simulink model "ModeloControlador2"  (R2018a)
settings: Solver=VariableStepAuto  StartTime=0.0  StopTime=20  RelTol=1e-3
values from neighbouring files (symbols this model uses):
  grav = 9.81    [modelodrone.m]
  Jr = .00006    (= 6e-05)    [modelodrone.m]
  massa = 1.24706    [modelodrone.m]
undefined symbols (not defined in the file or in its folder): Drone
libraries: simulink x6
settings Model: Creator=lg07j  LastModifiedBy=lg07j

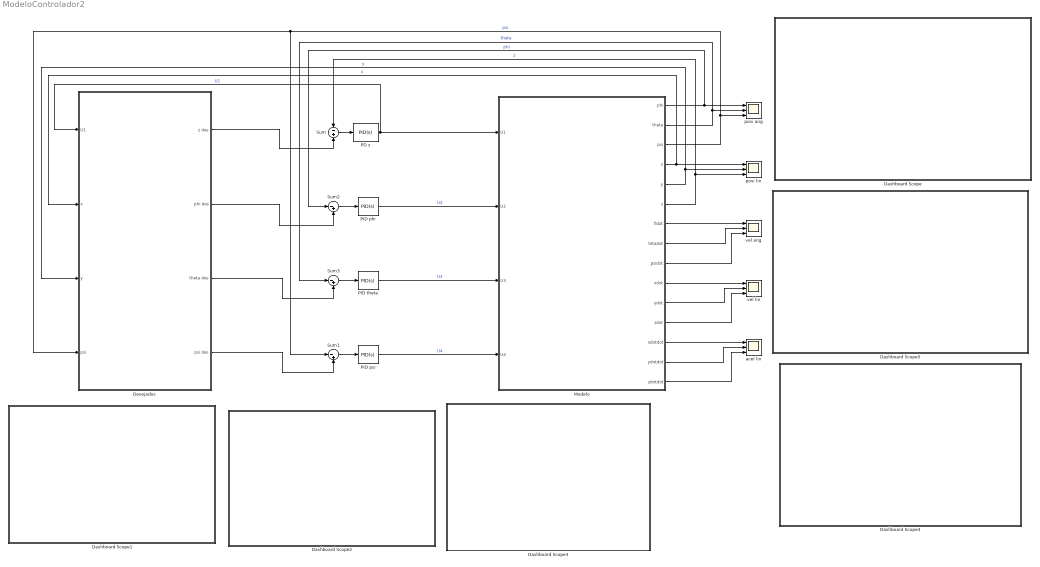
== system ModeloControlador2 ==
  Dashboard Scope : Subsystem  DialogController=hmiCreateDDGDialog  IsWebBlock=on  mask(MWDashboardBlock){webBlockId=ccebd60a-0072-45fe-991e-5f1cde7eeb39, webBlockType=sdiscope, ShowInitialText=on, HMISrcModelName=ModeloControlador2}
      mask prompts: webBlockId "WebBlock Id"; webBlockType "WebBlock Type"; HMISrcModelName "Source Model"
      mask help: SimulinkHMI:dialogs:HMIScopeDialogDesc
      mask Help: helpview([docroot '/mapfiles/simulink.map'], 'hmi_scope')
      mask Display:
      | if strcmp(get_param(bdroot(gcb),'BlockDiagramType'), 'library')
      |     image([(matlabroot) '/toolbox/simulink/hmi/icons/DashboardScope.png']);
      | end
  Dashboard Scope1 : Subsystem  DialogController=hmiCreateDDGDialog  IsWebBlock=on  mask(MWDashboardBlock){webBlockId=5c128209-e94a-417c-b40b-eaa209d18782, webBlockType=sdiscope, ShowInitialText=on, HMISrcModelName=ModeloControlador2}
      mask prompts: webBlockId "WebBlock Id"; webBlockType "WebBlock Type"; HMISrcModelName "Source Model"
      mask help: SimulinkHMI:dialogs:HMIScopeDialogDesc
      mask Help: helpview([docroot '/mapfiles/simulink.map'], 'hmi_scope')
      mask Display:
      | if strcmp(get_param(bdroot(gcb),'BlockDiagramType'), 'library')
      |     image([(matlabroot) '/toolbox/simulink/hmi/icons/DashboardScope.png']);
      | end
  Dashboard Scope2 : Subsystem  DialogController=hmiCreateDDGDialog  IsWebBlock=on  mask(MWDashboardBlock){webBlockId=3c2bd112-e6fb-4389-a652-d4a52c948602, webBlockType=sdiscope, ShowInitialText=on, HMISrcModelName=ModeloControlador2}
      mask prompts: webBlockId "WebBlock Id"; webBlockType "WebBlock Type"; HMISrcModelName "Source Model"
      mask help: SimulinkHMI:dialogs:HMIScopeDialogDesc
      mask Help: helpview([docroot '/mapfiles/simulink.map'], 'hmi_scope')
      mask Display:
      | if strcmp(get_param(bdroot(gcb),'BlockDiagramType'), 'library')
      |     image([(matlabroot) '/toolbox/simulink/hmi/icons/DashboardScope.png']);
      | end
  Dashboard Scope3 : Subsystem  DialogController=hmiCreateDDGDialog  IsWebBlock=on  mask(MWDashboardBlock){webBlockId=80d6d028-651e-447f-a397-777ee9cde126, webBlockType=sdiscope, ShowInitialText=on, HMISrcModelName=ModeloControlador2}
      mask prompts: webBlockId "WebBlock Id"; webBlockType "WebBlock Type"; HMISrcModelName "Source Model"
      mask help: SimulinkHMI:dialogs:HMIScopeDialogDesc
      mask Help: helpview([docroot '/mapfiles/simulink.map'], 'hmi_scope')
      mask Display:
      | if strcmp(get_param(bdroot(gcb),'BlockDiagramType'), 'library')
      |     image([(matlabroot) '/toolbox/simulink/hmi/icons/DashboardScope.png']);
      | end
  Dashboard Scope4 : Subsystem  DialogController=hmiCreateDDGDialog  IsWebBlock=on  mask(MWDashboardBlock){webBlockId=8646fb84-920d-4198-92bb-6f16b9d3f7b0, webBlockType=sdiscope, ShowInitialText=on, HMISrcModelName=ModeloControlador2}
      mask prompts: webBlockId "WebBlock Id"; webBlockType "WebBlock Type"; HMISrcModelName "Source Model"
      mask help: SimulinkHMI:dialogs:HMIScopeDialogDesc
      mask Help: helpview([docroot '/mapfiles/simulink.map'], 'hmi_scope')
      mask Display:
      | if strcmp(get_param(bdroot(gcb),'BlockDiagramType'), 'library')
      |     image([(matlabroot) '/toolbox/simulink/hmi/icons/DashboardScope.png']);
      | end
  Dashboard Scope5 : Subsystem  DialogController=hmiCreateDDGDialog  IsWebBlock=on  mask(MWDashboardBlock){webBlockId=bbe5046a-50a3-4443-b963-3734f90851a3, webBlockType=sdiscope, ShowInitialText=on, HMISrcModelName=ModeloControlador2}
      mask prompts: webBlockId "WebBlock Id"; webBlockType "WebBlock Type"; HMISrcModelName "Source Model"
      mask help: SimulinkHMI:dialogs:HMIScopeDialogDesc
      mask Help: helpview([docroot '/mapfiles/simulink.map'], 'hmi_scope')
      mask Display:
      | if strcmp(get_param(bdroot(gcb),'BlockDiagramType'), 'library')
      |     image([(matlabroot) '/toolbox/simulink/hmi/icons/DashboardScope.png']);
      | end
  Desejados : Subsystem
  Modelo : Subsystem
  PD z : simulink/Continuous/PID Controller  Controller=PID  TimeDomain=Continuous-time  SampleTime=-1  IntegratorMethod=Forward Euler  FilterMethod=Forward Euler  Form=Parallel  UseFilter=on  ControllerParametersSource=internal  P=-82.2920900762788  I=-66.9206931824462  D=-24.7314823181759  N=2285.65595208321  InitialConditionSource=internal  InitialConditionForIntegrator=0  InitialConditionForFilter=0  ExternalReset=none  LimitOutput=off  UpperSaturationLimit=inf  LowerSaturationLimit=-inf  LinearizeAsGain=on  AntiWindupMode=clamping  Kb=1  TrackingMode=off  Kt=1  PParamMin=[]  PParamMax=[]  IParamMin=[]  IParamMax=[]  DParamMin=[]  DParamMax=[]  NParamMin=[]  NParamMax=[]  KbParamMin=[]  KbParamMax=[]  KtParamMin=[]  KtParamMax=[]  POutMin=[]  POutMax=[]  IOutMin=[]  IOutMax=[]  DOutMin=[]  DOutMax=[]  NOutMin=[]  NOutMax=[]  KbOutMin=[]  KbOutMax=[]  KtOutMin=[]  KtOutMax=[]  IntegratorOutMin=[]  IntegratorOutMax=[]  FilterOutMin=[]  FilterOutMax=[]  SumOutMin=[]  SumOutMax=[]  SumI1OutMin=[]  SumI1OutMax=[]  SumI2OutMin=[]  SumI2OutMax=[]  SumI3OutMin=[]  SumI3OutMax=[]  SumDOutMin=[]  SumDOutMax=[]  SaturationOutMin=[]  SaturationOutMax=[]  IntegratorContinuousStateAttributes=''  IntegratorStateMustResolveToSignalObject=off  IntegratorRTWStateStorageClass=Auto  FilterContinuousStateAttributes=''  FilterStateMustResolveToSignalObject=off  FilterRTWStateStorageClass=Auto  DifferentiatorICPrevScaledInput=0  DifferentiatorOutMin=[]  DifferentiatorOutMax=[]  FilterDiffOutCoefMin=[]  FilterDiffOutCoefMax=[]  SumDenOutMin=[]  SumDenOutMax=[]  SumNumOutMin=[]  SumNumOutMax=[]  ReciprocalOutMin=[]  ReciprocalOutMax=[]  DivideOutMin=[]  DivideOutMax=[]  TunerSelectOption=Transfer Function Based (PID Tuner App)
  PID phi : simulink/Continuous/PID Controller  Controller=PID  TimeDomain=Continuous-time  SampleTime=-1  IntegratorMethod=Forward Euler  FilterMethod=Forward Euler  Form=Parallel  UseFilter=on  ControllerParametersSource=internal  P=0.152452364134825  I=0.0197643611520207  D=0.261280210470045  N=2539.6177245369  InitialConditionSource=internal  InitialConditionForIntegrator=0  InitialConditionForFilter=0  ExternalReset=none  LimitOutput=off  UpperSaturationLimit=800  LowerSaturationLimit=-800  LinearizeAsGain=on  AntiWindupMode=clamping  Kb=1  TrackingMode=off  Kt=1  PParamMin=[]  PParamMax=[]  IParamMin=[]  IParamMax=[]  DParamMin=[]  DParamMax=[]  NParamMin=[]  NParamMax=[]  KbParamMin=[]  KbParamMax=[]  KtParamMin=[]  KtParamMax=[]  POutMin=[]  POutMax=[]  IOutMin=[]  IOutMax=[]  DOutMin=[]  DOutMax=[]  NOutMin=[]  NOutMax=[]  KbOutMin=[]  KbOutMax=[]  KtOutMin=[]  KtOutMax=[]  IntegratorOutMin=[]  IntegratorOutMax=[]  FilterOutMin=[]  FilterOutMax=[]  SumOutMin=[]  SumOutMax=[]  SumI1OutMin=[]  SumI1OutMax=[]  SumI2OutMin=[]  SumI2OutMax=[]  SumI3OutMin=[]  SumI3OutMax=[]  SumDOutMin=[]  SumDOutMax=[]  SaturationOutMin=[]  SaturationOutMax=[]  IntegratorContinuousStateAttributes=''  IntegratorStateMustResolveToSignalObject=off  IntegratorRTWStateStorageClass=Auto  FilterContinuousStateAttributes=''  FilterStateMustResolveToSignalObject=off  FilterRTWStateStorageClass=Auto  DifferentiatorICPrevScaledInput=0  DifferentiatorOutMin=[]  DifferentiatorOutMax=[]  FilterDiffOutCoefMin=[]  FilterDiffOutCoefMax=[]  SumDenOutMin=[]  SumDenOutMax=[]  SumNumOutMin=[]  SumNumOutMax=[]  ReciprocalOutMin=[]  ReciprocalOutMax=[]  DivideOutMin=[]  DivideOutMax=[]  TunerSelectOption=Transfer Function Based (PID Tuner App)
  PID psi : simulink/Continuous/PID Controller  Controller=PID  TimeDomain=Continuous-time  SampleTime=-1  IntegratorMethod=Forward Euler  FilterMethod=Forward Euler  Form=Parallel  UseFilter=on  ControllerParametersSource=internal  P=0.222013595655969  I=0.0360989822121643  D=0.157215356027355  N=761.885317361069  InitialConditionSource=internal  InitialConditionForIntegrator=0  InitialConditionForFilter=0  ExternalReset=none  LimitOutput=off  UpperSaturationLimit=800  LowerSaturationLimit=-800  LinearizeAsGain=on  AntiWindupMode=none  Kb=1  TrackingMode=off  Kt=1  PParamMin=[]  PParamMax=[]  IParamMin=[]  IParamMax=[]  DParamMin=[]  DParamMax=[]  NParamMin=[]  NParamMax=[]  KbParamMin=[]  KbParamMax=[]  KtParamMin=[]  KtParamMax=[]  POutMin=[]  POutMax=[]  IOutMin=[]  IOutMax=[]  DOutMin=[]  DOutMax=[]  NOutMin=[]  NOutMax=[]  KbOutMin=[]  KbOutMax=[]  KtOutMin=[]  KtOutMax=[]  IntegratorOutMin=[]  IntegratorOutMax=[]  FilterOutMin=[]  FilterOutMax=[]  SumOutMin=[]  SumOutMax=[]  SumI1OutMin=[]  SumI1OutMax=[]  SumI2OutMin=[]  SumI2OutMax=[]  SumI3OutMin=[]  SumI3OutMax=[]  SumDOutMin=[]  SumDOutMax=[]  SaturationOutMin=[]  SaturationOutMax=[]  IntegratorContinuousStateAttributes=''  IntegratorStateMustResolveToSignalObject=off  IntegratorRTWStateStorageClass=Auto  FilterContinuousStateAttributes=''  FilterStateMustResolveToSignalObject=off  FilterRTWStateStorageClass=Auto  DifferentiatorICPrevScaledInput=0  DifferentiatorOutMin=[]  DifferentiatorOutMax=[]  FilterDiffOutCoefMin=[]  FilterDiffOutCoefMax=[]  SumDenOutMin=[]  SumDenOutMax=[]  SumNumOutMin=[]  SumNumOutMax=[]  ReciprocalOutMin=[]  ReciprocalOutMax=[]  DivideOutMin=[]  DivideOutMax=[]  TunerSelectOption=Transfer Function Based (PID Tuner App)
  PID theta : simulink/Continuous/PID Controller  Controller=PID  TimeDomain=Continuous-time  SampleTime=-1  IntegratorMethod=Forward Euler  FilterMethod=Forward Euler  Form=Parallel  UseFilter=on  ControllerParametersSource=internal  P=0.157396015622345  I=0.020405270290843  D=0.269752878693198  N=2539.6177245369  InitialConditionSource=internal  InitialConditionForIntegrator=0  InitialConditionForFilter=0  ExternalReset=none  LimitOutput=off  UpperSaturationLimit=800  LowerSaturationLimit=-800  LinearizeAsGain=on  AntiWindupMode=none  Kb=1  TrackingMode=off  Kt=1  PParamMin=[]  PParamMax=[]  IParamMin=[]  IParamMax=[]  DParamMin=[]  DParamMax=[]  NParamMin=[]  NParamMax=[]  KbParamMin=[]  KbParamMax=[]  KtParamMin=[]  KtParamMax=[]  POutMin=[]  POutMax=[]  IOutMin=[]  IOutMax=[]  DOutMin=[]  DOutMax=[]  NOutMin=[]  NOutMax=[]  KbOutMin=[]  KbOutMax=[]  KtOutMin=[]  KtOutMax=[]  IntegratorOutMin=[]  IntegratorOutMax=[]  FilterOutMin=[]  FilterOutMax=[]  SumOutMin=[]  SumOutMax=[]  SumI1OutMin=[]  SumI1OutMax=[]  SumI2OutMin=[]  SumI2OutMax=[]  SumI3OutMin=[]  SumI3OutMax=[]  SumDOutMin=[]  SumDOutMax=[]  SaturationOutMin=[]  SaturationOutMax=[]  IntegratorContinuousStateAttributes=''  IntegratorStateMustResolveToSignalObject=off  IntegratorRTWStateStorageClass=Auto  FilterContinuousStateAttributes=''  FilterStateMustResolveToSignalObject=off  FilterRTWStateStorageClass=Auto  DifferentiatorICPrevScaledInput=0  DifferentiatorOutMin=[]  DifferentiatorOutMax=[]  FilterDiffOutCoefMin=[]  FilterDiffOutCoefMax=[]  SumDenOutMin=[]  SumDenOutMax=[]  SumNumOutMin=[]  SumNumOutMax=[]  ReciprocalOutMin=[]  ReciprocalOutMax=[]  DivideOutMin=[]  DivideOutMax=[]  TunerSelectOption=Transfer Function Based (PID Tuner App)
  Sum : Sum  Inputs=-+
  Sum1 : Sum  Inputs=|-+
  Sum2 : Sum  Inputs=|-+
  Sum3 : Sum  Inputs=|-+
  acel lin : Scope  NumInputPorts=3
  posi ang : Scope  NumInputPorts=3
  posi lin : Scope  NumInputPorts=3
  vel ang : Scope  NumInputPorts=3
  vel lin : Scope  NumInputPorts=3
  wires:
  Modelo/1(phi) -> Sum2/1, posi ang/1  "phi"
  Modelo/2(theta) -> Sum3/1, posi ang/2  "theta"
  Modelo/3(psi) -> Desejados/4(psi), Sum1/1, posi ang/3  "psi"
  Modelo/4(x) -> Desejados/2(x), posi lin/1  "x"
  Modelo/5(y) -> posi lin/2, Desejados/3(y)  "y"
  Modelo/6(z) -> Sum/1, posi lin/3  "z"
  Modelo/7(fidot) -> vel ang/1
  Modelo/8(tetadot) -> vel ang/2
  Modelo/9(psidot) -> vel ang/3
  Modelo/11(ydot) -> vel lin/2
  Modelo/12(zdot) -> vel lin/3
  Modelo/14(ydotdot) -> acel lin/2
  Modelo/15(zdotdot) -> acel lin/3
  Modelo/10(xdot) -> vel lin/1
  Modelo/13(xdotdot) -> acel lin/1
  PID theta/1 -> Modelo/3(U3)  "U3"
  Sum1/1 -> PID psi/1
  PID psi/1 -> Modelo/4(U4)  "U4"
  PID phi/1 -> Modelo/2(U2)  "U2"
  Sum/1 -> PD z/1
  Sum2/1 -> PID phi/1
  Sum3/1 -> PID theta/1
  PD z/1 -> Desejados/1(U1), Modelo/1(U1)  "U1"
  Desejados/1(z des) -> Sum/2
  Desejados/2(phi des) -> Sum2/2
  Desejados/3(theta des) -> Sum3/2
  Desejados/4(psi des) -> Sum1/2

== system ModeloControlador2/Dashboard Scope ==

== system ModeloControlador2/Dashboard Scope1 ==

== system ModeloControlador2/Dashboard Scope2 ==

== system ModeloControlador2/Dashboard Scope3 ==

== system ModeloControlador2/Dashboard Scope4 ==

== system ModeloControlador2/Dashboard Scope5 ==

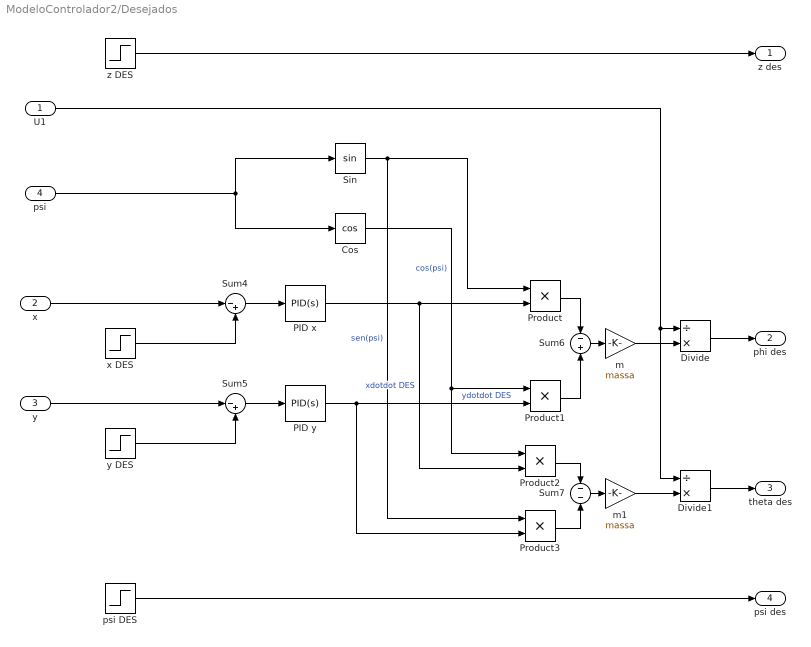
== system ModeloControlador2/Desejados ==
  U1 : Inport
  x : Inport  Port=2
  y : Inport  Port=3
  psi : Inport  Port=4
  Cos : Trigonometry  Operator=cos
  Divide : Product  Inputs=/*
  Divide1 : Product  Inputs=/*
  PID x : simulink/Continuous/PID Controller  Controller=PID  TimeDomain=Continuous-time  SampleTime=-1  IntegratorMethod=Forward Euler  FilterMethod=Forward Euler  Form=Parallel  UseFilter=on  ControllerParametersSource=internal  P=16.500836686522  I=6.7113771973829  D=9.91582425446305  N=1142.8279760416  InitialConditionSource=internal  InitialConditionForIntegrator=0  InitialConditionForFilter=0  ExternalReset=none  LimitOutput=off  UpperSaturationLimit=inf  LowerSaturationLimit=-inf  LinearizeAsGain=on  AntiWindupMode=none  Kb=1  TrackingMode=off  Kt=1  PParamMin=[]  PParamMax=[]  IParamMin=[]  IParamMax=[]  DParamMin=[]  DParamMax=[]  NParamMin=[]  NParamMax=[]  KbParamMin=[]  KbParamMax=[]  KtParamMin=[]  KtParamMax=[]  POutMin=[]  POutMax=[]  IOutMin=[]  IOutMax=[]  DOutMin=[]  DOutMax=[]  NOutMin=[]  NOutMax=[]  KbOutMin=[]  KbOutMax=[]  KtOutMin=[]  KtOutMax=[]  IntegratorOutMin=[]  IntegratorOutMax=[]  FilterOutMin=[]  FilterOutMax=[]  SumOutMin=[]  SumOutMax=[]  SumI1OutMin=[]  SumI1OutMax=[]  SumI2OutMin=[]  SumI2OutMax=[]  SumI3OutMin=[]  SumI3OutMax=[]  SumDOutMin=[]  SumDOutMax=[]  SaturationOutMin=[]  SaturationOutMax=[]  IntegratorContinuousStateAttributes=''  IntegratorStateMustResolveToSignalObject=off  IntegratorRTWStateStorageClass=Auto  FilterContinuousStateAttributes=''  FilterStateMustResolveToSignalObject=off  FilterRTWStateStorageClass=Auto  DifferentiatorICPrevScaledInput=0  DifferentiatorOutMin=[]  DifferentiatorOutMax=[]  FilterDiffOutCoefMin=[]  FilterDiffOutCoefMax=[]  SumDenOutMin=[]  SumDenOutMax=[]  SumNumOutMin=[]  SumNumOutMax=[]  ReciprocalOutMin=[]  ReciprocalOutMax=[]  DivideOutMin=[]  DivideOutMax=[]  TunerSelectOption=Transfer Function Based (PID Tuner App)
  PID y : simulink/Continuous/PID Controller  Controller=PID  TimeDomain=Continuous-time  SampleTime=-1  IntegratorMethod=Forward Euler  FilterMethod=Forward Euler  Form=Parallel  UseFilter=on  ControllerParametersSource=internal  P=16.4994310577233  I=6.70999951086392  D=9.91586568066273  N=1142.8279760416  InitialConditionSource=internal  InitialConditionForIntegrator=0  InitialConditionForFilter=0  ExternalReset=none  LimitOutput=off  UpperSaturationLimit=inf  LowerSaturationLimit=-inf  LinearizeAsGain=on  AntiWindupMode=none  Kb=1  TrackingMode=off  Kt=1  PParamMin=[]  PParamMax=[]  IParamMin=[]  IParamMax=[]  DParamMin=[]  DParamMax=[]  NParamMin=[]  NParamMax=[]  KbParamMin=[]  KbParamMax=[]  KtParamMin=[]  KtParamMax=[]  POutMin=[]  POutMax=[]  IOutMin=[]  IOutMax=[]  DOutMin=[]  DOutMax=[]  NOutMin=[]  NOutMax=[]  KbOutMin=[]  KbOutMax=[]  KtOutMin=[]  KtOutMax=[]  IntegratorOutMin=[]  IntegratorOutMax=[]  FilterOutMin=[]  FilterOutMax=[]  SumOutMin=[]  SumOutMax=[]  SumI1OutMin=[]  SumI1OutMax=[]  SumI2OutMin=[]  SumI2OutMax=[]  SumI3OutMin=[]  SumI3OutMax=[]  SumDOutMin=[]  SumDOutMax=[]  SaturationOutMin=[]  SaturationOutMax=[]  IntegratorContinuousStateAttributes=''  IntegratorStateMustResolveToSignalObject=off  IntegratorRTWStateStorageClass=Auto  FilterContinuousStateAttributes=''  FilterStateMustResolveToSignalObject=off  FilterRTWStateStorageClass=Auto  DifferentiatorICPrevScaledInput=0  DifferentiatorOutMin=[]  DifferentiatorOutMax=[]  FilterDiffOutCoefMin=[]  FilterDiffOutCoefMax=[]  SumDenOutMin=[]  SumDenOutMax=[]  SumNumOutMin=[]  SumNumOutMax=[]  ReciprocalOutMin=[]  ReciprocalOutMax=[]  DivideOutMin=[]  DivideOutMax=[]  TunerSelectOption=Transfer Function Based (PID Tuner App)
  Product{,1..3} (4 alike) : Product
  Sin : Trigonometry
  Sum4 : Sum  Inputs=|-+
  Sum5 : Sum  Inputs=|-+
  Sum6 : Sum  Inputs=-+
  Sum7 : Sum  Inputs=--
  m : Gain  Gain=massa
  m1 : Gain  Gain=massa
  psi DES : Step  Time=0  SampleTime=0
  "x DES " : Step  Time=0  SampleTime=0
  y DES : Step  Time=0  SampleTime=0
  z DES : Step  Time=0  SampleTime=0
  z des : Outport
  phi des : Outport  Port=2
  theta des : Outport  Port=3
  psi des : Outport  Port=4
  wires:
  y DES/1 -> Sum5/2
  Cos/1 -> Product2/1, Product1/1  "cos(psi)"
  Sin/1 -> Product3/1, Product/1  "sen(psi)"
  "x DES "/1 -> Sum4/2
  Product/1 -> Sum6/1
  U1/1 -> Divide1/1, Divide/1
  Sum6/1 -> m/1
  PID y/1 -> Product3/2, Product1/2  "ydotdot DES"
  Product3/1 -> Sum7/2
  psi/1 -> Sin/1, Cos/1
  m/1 -> Divide/2
  Product1/1 -> Sum6/2
  Sum5/1 -> PID y/1
  Sum4/1 -> PID x/1
  Product2/1 -> Sum7/1
  m1/1 -> Divide1/2
  Sum7/1 -> m1/1
  PID x/1 -> Product/2, Product2/2  "xdotdot DES"
  Divide/1 -> phi des/1
  psi DES/1 -> psi des/1
  z DES/1 -> z des/1
  Divide1/1 -> theta des/1
  x/1 -> Sum4/1
  y/1 -> Sum5/1

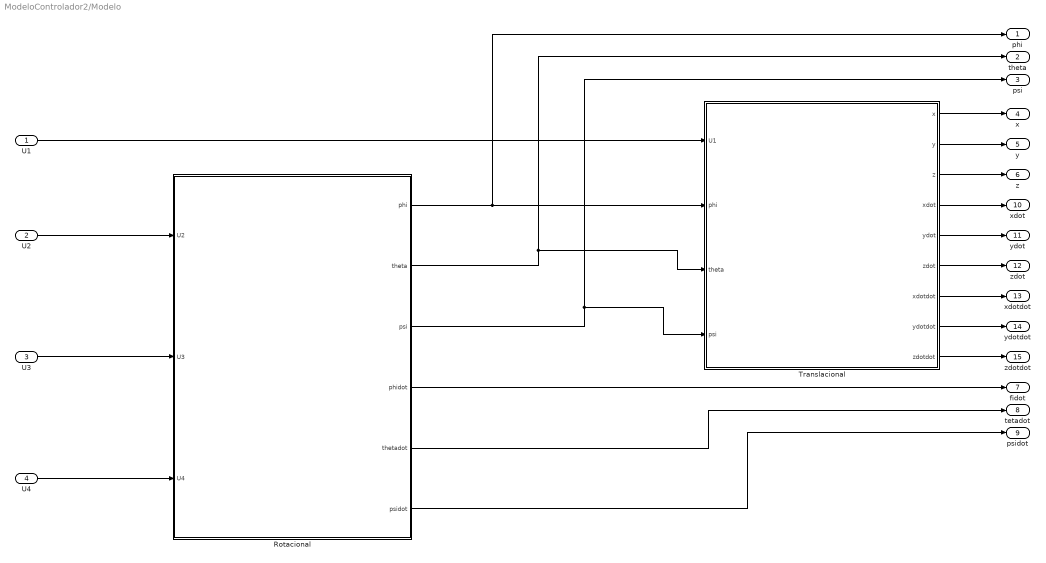
== system ModeloControlador2/Modelo ==
  U1 : Inport
  U2 : Inport  Port=2
  U3 : Inport  Port=3
  U4 : Inport  Port=4
  Rotacional : Subsystem
  Translacional : Subsystem
  phi : Outport
  theta : Outport  Port=2
  psi : Outport  Port=3
  x : Outport  Port=4
  y : Outport  Port=5
  z : Outport  Port=6
  fidot : Outport  Port=7
  tetadot : Outport  Port=8
  psidot : Outport  Port=9
  xdot : Outport  Port=10
  ydot : Outport  Port=11
  zdot : Outport  Port=12
  xdotdot : Outport  Port=13
  ydotdot : Outport  Port=14
  zdotdot : Outport  Port=15
  wires:
  Rotacional/2(theta) -> Translacional/3(theta), theta/1
  Rotacional/6(psidot) -> psidot/1
  Rotacional/1(phi) -> phi/1, Translacional/2(phi)
  Rotacional/4(phidot) -> fidot/1
  Rotacional/3(psi) -> Translacional/4(psi), psi/1
  Rotacional/5(thetadot) -> tetadot/1
  Translacional/4(xdot) -> xdot/1
  Translacional/3(z) -> z/1
  Translacional/8(ydotdot) -> ydotdot/1
  Translacional/5(ydot) -> ydot/1
  U3/1 -> Rotacional/2(U3)
  U1/1 -> Translacional/1(U1)
  U4/1 -> Rotacional/3(U4)
  Translacional/1(x) -> x/1
  U2/1 -> Rotacional/1(U2)
  Translacional/7(xdotdot) -> xdotdot/1
  Translacional/2(y) -> y/1
  Translacional/9(zdotdot) -> zdotdot/1
  Translacional/6(zdot) -> zdot/1

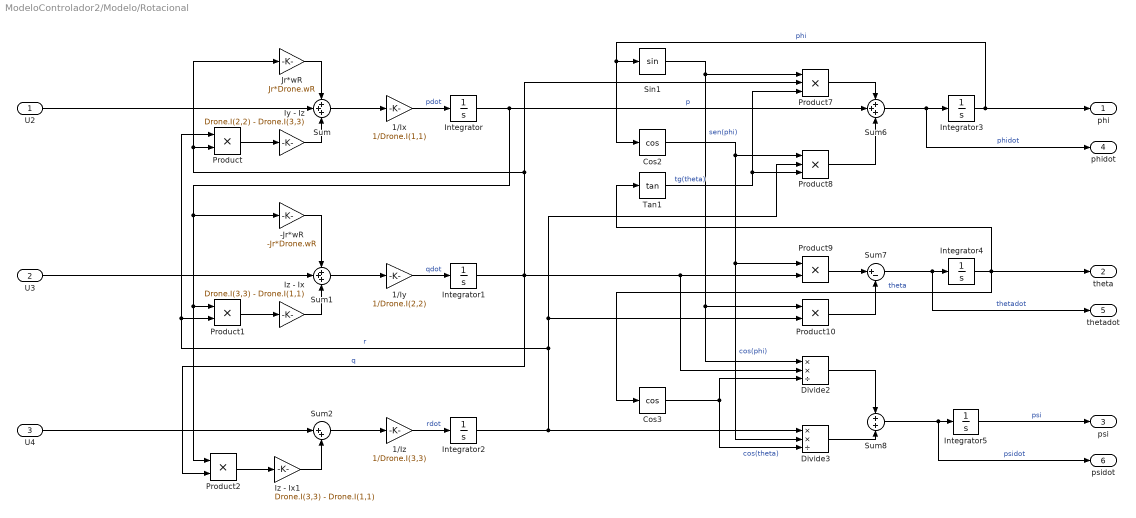
== system ModeloControlador2/Modelo/Rotacional ==
  U2 : Inport
  U3 : Inport  Port=2
  U4 : Inport  Port=3
  -Jr*wR : Gain  Gain=-Jr*Drone.wR
  1/Ix : Gain  Gain=1/Drone.I(1,1)
  1/Iy : Gain  Gain=1/Drone.I(2,2)
  1/Iz : Gain  Gain=1/Drone.I(3,3)
  Cos2 : Trigonometry  Operator=cos
  Cos3 : Trigonometry  Operator=cos
  Divide2 : Product  Inputs=**/
  Divide3 : Product  Inputs=**/
  Integrator{,1..5} (6 alike) : Integrator
  Iy - Iz : Gain  Gain=Drone.I(2,2) - Drone.I(3,3)
  Iz - Ix : Gain  Gain=Drone.I(3,3) - Drone.I(1,1)
  Iz - Ix1 : Gain  Gain=Drone.I(3,3) - Drone.I(1,1)
  Jr*wR : Gain  Gain=Jr*Drone.wR
  Product{,1..2,9..10} (5 alike) : Product
  Product7 : Product  Inputs=3
  Product8 : Product  Inputs=3
  Sin1 : Trigonometry
  Sum : Sum  Inputs=+++
  Sum1 : Sum  Inputs=+++
  Sum2 : Sum  Inputs=|++
  Sum6 : Sum  Inputs=+++
  Sum7 : Sum  Inputs=|+-
  Sum8 : Sum
  Tan1 : Trigonometry  Operator=tan
  phi : Outport
  theta : Outport  Port=2
  psi : Outport  Port=3
  phidot : Outport  Port=4
  thetadot : Outport  Port=5
  psidot : Outport  Port=6
  wires:
  1/Ix/1 -> Integrator/1  "pdot"
  Sum1/1 -> 1/Iy/1
  1/Iz/1 -> Integrator2/1  "rdot"
  Sum/1 -> 1/Ix/1
  U2/1 -> Sum/2
  Iy - Iz/1 -> Sum/3
  Product/1 -> Iy - Iz/1
  Jr*wR/1 -> Sum/1
  -Jr*wR/1 -> Sum1/1
  U3/1 -> Sum1/2
  Product1/1 -> Iz - Ix/1
  Iz - Ix/1 -> Sum1/3
  1/Iy/1 -> Integrator1/1  "qdot"
  Sum2/1 -> 1/Iz/1
  U4/1 -> Sum2/1
  Product2/1 -> Iz - Ix1/1
  Iz - Ix1/1 -> Sum2/2
  Integrator5/1 -> psi/1  "psi"
  Cos3/1 -> Divide3/3, Divide2/3  "cos(theta)"
  Divide2/1 -> Sum8/1
  Product8/1 -> Sum6/3
  Integrator3/1 -> Cos2/1, Sin1/1, phi/1  "phi"
  Product9/1 -> Sum7/1
  Cos2/1 -> Divide3/2, Product9/1, Product8/1  "cos(phi)"
  Sum7/1 -> Integrator4/1, thetadot/1  "thetadot"
  Divide3/1 -> Sum8/2
  Product10/1 -> Sum7/2
  Product7/1 -> Sum6/1
  Sum6/1 -> Integrator3/1, phidot/1  "phidot"
  Integrator2/1 -> Divide3/1, Product10/2, Product8/2, Product1/2, Product/1  "r"
  Tan1/1 -> Product7/3, Product8/3  "tg(theta)"
  Sum8/1 -> Integrator5/1, psidot/1  "psidot"
  Sin1/1 -> Divide2/1, Product10/1, Product7/1  "sen(phi)"
  Integrator/1 -> Sum6/2, -Jr*wR/1, Product2/1, Product1/1  "p"
  Integrator4/1 -> Cos3/1, Tan1/1, theta/1  "theta"
  Integrator1/1 -> Divide2/2, Product9/2, Product7/2, Jr*wR/1, Product/2, Product2/2  "q"

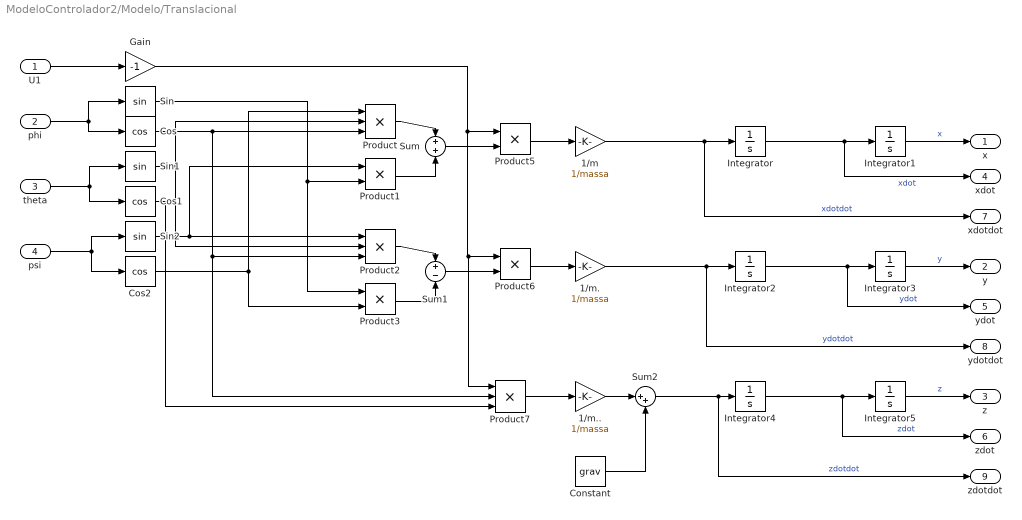
== system ModeloControlador2/Modelo/Translacional ==
  U1 : Inport
  phi : Inport  Port=2
  theta : Inport  Port=3
  psi : Inport  Port=4
  1/m : Gain  Gain=1/massa
  1/m. : Gain  Gain=1/massa
  1/m.. : Gain  Gain=1/massa
  Constant : Constant  Value=grav
  Cos : Trigonometry  Operator=cos
  Cos1 : Trigonometry  Operator=cos
  Cos2 : Trigonometry  Operator=cos
  Gain : Gain  Gain=-1
  Integrator{,1..5} (6 alike) : Integrator
  Product : Product  Inputs=3
  Product{1,3,5..6} (4 alike) : Product
  Product2 : Product  Inputs=3
  Product7 : Product  Inputs=3
  Sin : Trigonometry
  Sin1 : Trigonometry
  Sin2 : Trigonometry
  Sum : Sum
  Sum1 : Sum  Inputs=+-
  Sum2 : Sum  Inputs=|++
  x : Outport
  y : Outport  Port=2
  z : Outport  Port=3
  xdot : Outport  Port=4
  ydot : Outport  Port=5
  zdot : Outport  Port=6
  xdotdot : Outport  Port=7
  ydotdot : Outport  Port=8
  zdotdot : Outport  Port=9
  wires:
  Sum2/1 -> zdotdot/1, Integrator4/1  "zdotdot"
  Product2/1 -> Sum1/1
  Product/1 -> Sum/1
  Product1/1 -> Sum/2
  Integrator3/1 -> y/1  "y"
  Product5/1 -> 1/m/1
  phi/1 -> Sin/1, Cos/1
  Sin2/1 -> Product1/1, Product2/1
  Sum/1 -> Product5/2
  Product3/1 -> Sum1/2
  Constant/1 -> Sum2/2
  psi/1 -> Sin2/1, Cos2/1
  Cos2/1 -> Product/1, Product3/2
  1/m/1 -> xdotdot/1, Integrator/1  "xdotdot"
  Sum1/1 -> Product6/2
  Cos1/1 -> Product7/3
  Product7/1 -> 1/m../1
  Integrator4/1 -> zdot/1, Integrator5/1  "zdot"
  Integrator1/1 -> x/1  "x"
  1/m../1 -> Sum2/1
  Integrator/1 -> xdot/1, Integrator1/1  "xdot"
  1/m./1 -> ydotdot/1, Integrator2/1  "ydotdot"
  Integrator2/1 -> ydot/1, Integrator3/1  "ydot"
  Integrator5/1 -> z/1  "z"
  U1/1 -> Gain/1
  Product6/1 -> 1/m./1
  Gain/1 -> Product7/1, Product6/1, Product5/1
  theta/1 -> Sin1/1, Cos1/1
  Cos/1 -> Product7/2, Product2/3, Product/3
  Sin/1 -> Product1/2, Product3/1
  Sin1/1 -> Product2/2, Product/2
